simulink model "RM3_Hydraulic_PTO_NEW"  (R2019b)
settings: Solver=ode14x  StartTime=0  StopTime=200  FixedStep=0.0025  MaxStep=0.0025  RelTol=1e-3  EnableMultiTasking=on
undefined symbols (not defined in the file or in its folder): body, DiscIntNeverNeededParam, pto
libraries: fl_lib x1519, nesl_utility x807, sh_lib x675, WECSim_Lib x5
(part 2 of 56)

== system RM3_Hydraulic_PTO_NEW/PTO-Sim - Crankshaft DA 4 Cylinders Case 2 extra ==
  response : Inport
  " Flow Rate Accum Sensor" : fl_lib/Hydraulic/Hydraulic Sensors/Hydraulic Flow Rate Sensor  Commented=on
      settings: SourceProductName=Simscape
  1000 psi Pressure Relief Valve : sh_lib/Valves/Pressure Control Valves/Pressure Relief Valve  valve_area_spec=1  p_diff_TLU=[30.15e5 : 15e3 : 31.35e5] Pa  area_TLU=[1 : 1 : 9] .* 1e-5 m^2  area_max=pi*(0.75/2)^2 in^2  pres_set=1000 psi  reg_range=50 psi  C_d=0.7  A_leak=1e-12 m^2  lam_spec=1  B_lam=0.999  Re_cr=12  dynamic=0  tau=0.1 s  area_init=1e-12 m^2
      settings: SourceProductName=Simscape Fluids  SourceProductBaseCode=SH  InternalSimscapePortConfiguration="{\"Bottom\":[],\"Left\":[{\"id\":\"A\",\"label\":\"A\",\"type\":\"foundation.hydraulic.hydraulic\"}],\"Right\":[{\"id\":\"B\",\"label\":\"B\",\"type\":\"foundation.hydraulic.hydraulic\"}],\"Top\":[]}"
  Accumulator Volume Scope : Scope  Commented=on
  Ang Velocity signal : Product  Inputs=*/
  Bus Selector : BusSelector  OutputSignals=position,velocity
  Constant1 : Constant  Value=0
  Crank Initial Angle (rad) 1 : Constant  Value=pi/2
  Crank Initial Angle (rad) 2 : Constant  Value=0
  Crank Initial Angle (rad) 3 : Constant  Value=3*pi/2
  Crank Initial Angle (rad) 4 : Constant  Value=pi
  Crank Radius (m) : Constant  Value=0.1397
  Cylinder 1 : Subsystem
  Cylinder 2 : Subsystem
  Cylinder 3 : Subsystem
  Cylinder 4 : Subsystem
  Delay1 : Delay  Commented=on  DelayLength=1
  Delay2 : Delay  DelayLength=1
  Discrete-Time Integrator : DiscreteIntegrator  Commented=on  SampleTime=-1  ICPrevOutput=DiscIntNeverNeededParam  ICPrevScaledInput=DiscIntNeverNeededParam
  Discrete-Time Integrator - Angle Disp : DiscreteIntegrator  SampleTime=-1  ICPrevOutput=DiscIntNeverNeededParam  ICPrevScaledInput=DiscIntNeverNeededParam
  Gain : Gain  Commented=on
  Gain1 : Gain  Commented=on  Gain=-11000
  Gas-Charged Accumulator : sh_lib/Accumulators/Gas-Charged Accumulator  Commented=on  capacity=2.5 gal  dead_volume=4e-5 m^3  pr_preload=800 psi  k_sh=1.4  stiff_coeff=1e10 Pa/m^3  penetr_coeff=1e10 s*Pa/m^6  flow_rate_specify=off  flow_rate_priority=None  flow_rate=0.005 m^3/s  flow_rate_nominal_specify=off  flow_rate_nominal_unit=m^3/s  flow_rate_nominal_value=1  liquid_volume_specify=on  liquid_volume_priority=High  liquid_volume=0.005 m^3  liquid_volume_nominal_specify=off  liquid_volume_nominal_unit=m^3  liquid_volume_nominal_value=1  liquid_pressure_specify=off  liquid_pressure_priority=None  liquid_pressure=1.01325e+5 Pa  liquid_pressure_nominal_specify=off  liquid_pressure_nominal_unit=Pa  liquid_pressure_nominal_value=1
      settings: SourceProductName=Simscape Fluids  SourceProductBaseCode=SH  InternalSimscapePortConfiguration="{\"Bottom\":[],\"Left\":[],\"Right\":[{\"id\":\"A\",\"label\":\"A\",\"type\":\"foundation.hydraulic.hydraulic\"}],\"Top\":[]}"
  Hydraulic Reference : fl_lib/Hydraulic/Hydraulic Elements/Hydraulic Reference
      settings: SourceProductName=Simscape
  Ideal Angular Velocity Source : fl_lib/Mechanical/Mechanical Sources/Ideal Angular Velocity Source
  Linear Position Scope : Scope
  Linear Velocity Scope : Scope
  Mechanical Rotational Reference : fl_lib/Mechanical/Rotational Elements/Mechanical Rotational Reference
  Mux : Mux  Inputs=10
  Mux1 : Mux  Inputs=3
  Ocean Intake (5m depth) : fl_lib/Hydraulic/Hydraulic Elements/Hydraulic Reference
      settings: SourceProductName=Simscape
  PS-Simulink Converter : nesl_utility/PS-Simulink Converter  Commented=on  PhysicalDomain=network_engine_domain  SubClassName=ps_output  LeftPortType=input  RightPortType=output  PseudoPeriodic=off  Frequencies=[]  Unit=inherit  AffineConversion=off
  PS-Simulink Converter{1..10} (10 alike) : nesl_utility/PS-Simulink Converter  PhysicalDomain=network_engine_domain  SubClassName=ps_output  LeftPortType=input  RightPortType=output  PseudoPeriodic=off  Frequencies=[]  Unit=inherit  AffineConversion=off
  Plus : Sum  Commented=on
  "Point of zero spring force (submerged distance) " : Constant  Value=4
  Pressure Sensor RV : fl_lib/Hydraulic/Hydraulic Sensors/Hydraulic Pressure Sensor
      settings: SourceProductName=Simscape
  Product : Product
  RO Membrane : Subsystem
  Sea Water : sh_lib/Hydraulic Utilities/Hydraulic Fluid  DataSource=1  SelFluid=24  SysTemp=30  TrapAir=0.005  ViscDerFactor=1  range_error=2
      settings: SourceProductName=Simscape Fluids
  Selector : Selector  InputPortWidth=6  IndexOptions=Index vector (dialog)  Indices=3  OutputSizes=1
  Selector1 : Selector  InputPortWidth=6  IndexOptions=Index vector (dialog)  Indices=3  OutputSizes=1
  Simulink-PS Converter : nesl_utility/Simulink-PS Converter  PhysicalDomain=network_engine_domain  SubClassName=ps_input  LeftPortType=input  RightPortType=output  PseudoPeriodic=off  Frequencies=[]  NoiseDistribution=none  NoiseParameters=[]  Unit=rad/s  AffineConversion=off  FilteringAndDerivatives=filter  SimscapeFilterOrder=2  InputFilterTimeConstant=0.001  UdotUserProvided=0
  Sine Wave2 : Sin  Commented=on  Amplitude=0.45  Frequency=0.9  SampleTime=0.01
  Solver Configuration : nesl_utility/Solver Configuration  PhysicalDomain=network_engine_domain  SubClassName=solver  LeftPortType=input  RightPortType=generic  Tones=[]  Harmonics=[]  SimulateNoise=off  Profile=off  UseLocalSampling=off  EnableSwitchedLinearOptims=on  FrequencyDomain=off  UseCCode=off  RelTol=0.001  AbsTol=1e-06  MinStep=1e-09  ToWorkspace=off  RevertToSquareIcSolve=off  NumHomotopyIterations=100  PhasorMode=off  PhasorModeNumHarmonics=1  DoDC=off  ResidualTolerance=1e-09  UseLocalSolver=off  LocalSolverChoice=NE_BACKWARD_EULER_ADVANCER  LocalSolverSampleTime=0.001  DoFixedCost=off  MaxNonlinIter=3  MaxModeIter=2  LinearAlgebra=auto  EquationFormulation=NE_TIME_EF  DelaysMemoryBudget=1024  AutomaticFiltering=on  FilteringTimeConstant=0.01  PartitionStorageMethod=AS_NEEDED  PartitionMemoryBudget=1024  PartitionMethod=ROBUST
  Spool Radius (m) : Constant  Value=0.1397
  Spring Constant : Gain  Gain=-200
  Spring Constant1 : Gain  Commented=on  Gain=840
  Spring Constant2 : Gain  Commented=on  Gain=-400
  Sum : Sum  Inputs=|++
  Sum1 : Sum  Inputs=|++
  Sum2 : Sum  Inputs=4
  Switch : Switch  Criteria=u2 > Threshold
  Terminator : Terminator
  To Workspace : ToWorkspace  VariableName=output_RO  SaveFormat=Structure With Time  SampleTime=-1
  To Workspace1 : ToWorkspace  VariableName=output_Power  SaveFormat=Structure With Time  SampleTime=-1
  Water Quality Block : Subsystem
  Forces : Outport  VectorParamsAs1DForOutWhenUnconnected=off
  wires:
  Bus Selector/1 -> Selector/1  "<position>"
  Bus Selector/2 -> Selector1/1  "<velocity>"
  response/1 -> Bus Selector/1
  Selector/1 -> Linear Position Scope/1, Sum1/1, Terminator/1
  Spring Constant/1 -> Sum/2
  Gain1/1 -> Plus/2
  Sum/1 -> Delay2/1
  Constant1/1 -> Switch/3
  Switch/1 -> Ang Velocity signal/1
  Selector1/1 -> Linear Velocity Scope/1, Mux1/3, Product/1, Switch/2, Switch/1  "V_linear"
  Ang Velocity signal/1 -> Discrete-Time Integrator - Angle Disp/1, Simulink-PS Converter/1
  "Point of zero spring force (submerged distance) "/1 -> Sum1/2
  Sum1/1 -> Spring Constant/1
  Delay2/1 -> Product/2, Mux1/1, Forces/1  "Force"
  PS-Simulink Converter/1 -> Discrete-Time Integrator/1
  Discrete-Time Integrator/1 -> Accumulator Volume Scope/1
  Crank Radius (m)/1 -> Cylinder 4/1(Crank Radius), Cylinder 3/1(Crank Radius), Cylinder 2/1(Crank Radius), Cylinder 1/1(Crank Radius)
  Discrete-Time Integrator - Angle Disp/1 -> Cylinder 4/3(Angle Displacement), Cylinder 3/3(Angle Displacement), Cylinder 2/3(Angle Displacement), Cylinder 1/3(Angle Displacement)
  Crank Initial Angle (rad) 1/1 -> Cylinder 1/4(Crank Init Angle)
  Sum2/1 -> Sum/1
  Cylinder 1/1(PTO Force) -> Sum2/4
  Cylinder 2/1(PTO Force) -> Sum2/3
  Cylinder 3/1(PTO Force) -> Sum2/2
  Cylinder 4/1(PTO Force) -> Sum2/1
  Spool Radius (m)/1 -> Cylinder 1/2(Spool Radius), Cylinder 4/2(Spool Radius), Cylinder 3/2(Spool Radius), Cylinder 2/2(Spool Radius), Ang Velocity signal/2
  Crank Initial Angle (rad) 4/1 -> Cylinder 4/4(Crank Init Angle)
  Crank Initial Angle (rad) 3/1 -> Cylinder 3/4(Crank Init Angle)
  Crank Initial Angle (rad) 2/1 -> Cylinder 2/4(Crank Init Angle)
  PS-Simulink Converter6/1 -> Mux/7  "Feed Mass Flow Rate"
  PS-Simulink Converter10/1 -> Mux/6  "Brine Mass Flow Rate"
  PS-Simulink Converter9/1 -> Mux/9  "Brine Flow Rate"
  PS-Simulink Converter8/1 -> Mux/8  "Permeate Mass Flow Rate"
  Mux/1 -> To Workspace/1
  PS-Simulink Converter4/1 -> Mux/4  "Permeate Flow Rate"
  PS-Simulink Converter1/1 -> Mux/1  "P before RO after OSM"
  PS-Simulink Converter2/1 -> Mux/2  "P drop RO"
  PS-Simulink Converter3/1 -> Mux/3  "Feed Flow Rate"
  PS-Simulink Converter5/1 -> Mux/5  "Feed Pressure"
  PS-Simulink Converter7/1 -> Mux/10  "Pressure Brine Exit"
  Mux1/1 -> To Workspace1/1
  Product/1 -> Mux1/2  "Power"
  connections:
  Solver Configuration/RConn1 -- Ocean Intake (5m depth)/LConn1 -- Sea Water/RConn1 -- Cylinder 4/LConn3 -- Cylinder 3/LConn3 -- Cylinder 2/LConn3 -- Cylinder 1/LConn3
  Ideal Angular Velocity Source/RConn2 -- Mechanical Rotational Reference/LConn1
  Ideal Angular Velocity Source/RConn1 -- Simulink-PS Converter/RConn1
  1000 psi Pressure Relief Valve/RConn1 -- Pressure Sensor RV/RConn1 -- Hydraulic Reference/LConn1
  Gas-Charged Accumulator/RConn1 -- Cylinder 1/LConn2 -- Cylinder 3/LConn2 -- Cylinder 4/LConn2 -- Cylinder 2/LConn2 -- RO Membrane/LConn1 -- 1000 psi Pressure Relief Valve/LConn1 -- Pressure Sensor RV/LConn1
  " Flow Rate Accum Sensor"/RConn1 -- PS-Simulink Converter/LConn1
  Cylinder 1/LConn1 -- Cylinder 2/LConn1 -- Cylinder 3/LConn1 -- Cylinder 4/LConn1 -- Ideal Angular Velocity Source/LConn1
  PS-Simulink Converter10/LConn1 -- RO Membrane/RConn9
  PS-Simulink Converter3/LConn1 -- RO Membrane/RConn3 -- Water Quality Block/LConn3
  PS-Simulink Converter9/LConn1 -- RO Membrane/RConn8
  PS-Simulink Converter1/LConn1 -- RO Membrane/RConn1 -- Water Quality Block/LConn1
  PS-Simulink Converter8/LConn1 -- RO Membrane/RConn7
  PS-Simulink Converter6/LConn1 -- RO Membrane/RConn6
  RO Membrane/RConn4 -- PS-Simulink Converter4/LConn1 -- Water Quality Block/LConn4
  PS-Simulink Converter2/LConn1 -- RO Membrane/RConn2 -- Water Quality Block/LConn2
  RO Membrane/RConn5 -- PS-Simulink Converter5/LConn1
  PS-Simulink Converter7/LConn1 -- RO Membrane/RConn10

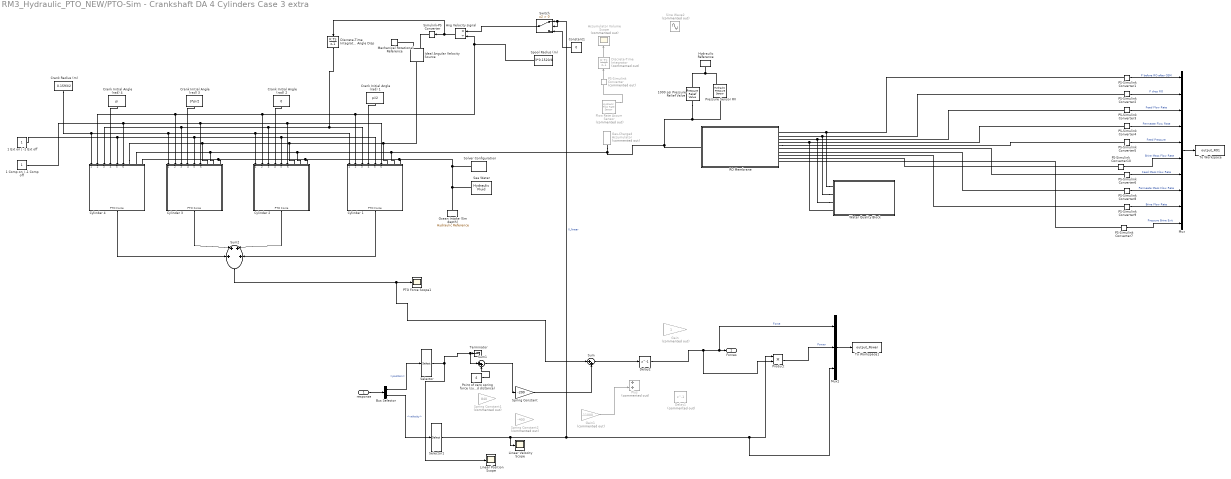
== system RM3_Hydraulic_PTO_NEW/PTO-Sim - Crankshaft DA 4 Cylinders Case 3 extra ==
  response : Inport
  " Flow Rate Accum Sensor" : fl_lib/Hydraulic/Hydraulic Sensors/Hydraulic Flow Rate Sensor  Commented=on
      settings: SourceProductName=Simscape
  1 Comp on | -1 Comp off : Constant
  1 Ext on | -1 Ext off : Constant
  1000 psi Pressure Relief Valve : sh_lib/Valves/Pressure Control Valves/Pressure Relief Valve  valve_area_spec=1  p_diff_TLU=[30.15e5 : 15e3 : 31.35e5] Pa  area_TLU=[1 : 1 : 9] .* 1e-5 m^2  area_max=pi*(0.75/2)^2 in^2  pres_set=1000 psi  reg_range=50 psi  C_d=0.7  A_leak=1e-12 m^2  lam_spec=1  B_lam=0.999  Re_cr=12  dynamic=0  tau=0.1 s  area_init=1e-12 m^2
      settings: SourceProductName=Simscape Fluids  SourceProductBaseCode=SH  InternalSimscapePortConfiguration="{\"Bottom\":[],\"Left\":[{\"id\":\"A\",\"label\":\"A\",\"type\":\"foundation.hydraulic.hydraulic\"}],\"Right\":[{\"id\":\"B\",\"label\":\"B\",\"type\":\"foundation.hydraulic.hydraulic\"}],\"Top\":[]}"
  Accumulator Volume Scope : Scope  Commented=on
  Ang Velocity signal : Product  Inputs=*/
  Bus Selector : BusSelector  OutputSignals=position,velocity
  Constant1 : Constant  Value=0
  Crank Initial Angle (rad) 1 : Constant  Value=pi/2
  Crank Initial Angle (rad) 2 : Constant  Value=0
  Crank Initial Angle (rad) 3 : Constant  Value=3*pi/2
  Crank Initial Angle (rad) 4 : Constant  Value=pi
  Crank Radius (m) : Constant  Value=0.1593/2
  Cylinder 1 : Subsystem
  Cylinder 2 : Subsystem
  Cylinder 3 : Subsystem
  Cylinder 4 : Subsystem
  Delay1 : Delay  Commented=on  DelayLength=1
  Delay2 : Delay  DelayLength=1
  Discrete-Time Integrator : DiscreteIntegrator  Commented=on  SampleTime=-1  ICPrevOutput=DiscIntNeverNeededParam  ICPrevScaledInput=DiscIntNeverNeededParam
  Discrete-Time Integrator - Angle Disp : DiscreteIntegrator  SampleTime=-1  ICPrevOutput=DiscIntNeverNeededParam  ICPrevScaledInput=DiscIntNeverNeededParam
  Gain : Gain  Commented=on
  Gain1 : Gain  Commented=on  Gain=-11000
  Gas-Charged Accumulator : sh_lib/Accumulators/Gas-Charged Accumulator  Commented=on  capacity=2.5 gal  dead_volume=4e-5 m^3  pr_preload=800 psi  k_sh=1.4  stiff_coeff=1e10 Pa/m^3  penetr_coeff=1e10 s*Pa/m^6  flow_rate_specify=off  flow_rate_priority=None  flow_rate=0.005 m^3/s  flow_rate_nominal_specify=off  flow_rate_nominal_unit=m^3/s  flow_rate_nominal_value=1  liquid_volume_specify=on  liquid_volume_priority=High  liquid_volume=0.005 m^3  liquid_volume_nominal_specify=off  liquid_volume_nominal_unit=m^3  liquid_volume_nominal_value=1  liquid_pressure_specify=off  liquid_pressure_priority=None  liquid_pressure=1.01325e+5 Pa  liquid_pressure_nominal_specify=off  liquid_pressure_nominal_unit=Pa  liquid_pressure_nominal_value=1
      settings: SourceProductName=Simscape Fluids  SourceProductBaseCode=SH  InternalSimscapePortConfiguration="{\"Bottom\":[],\"Left\":[],\"Right\":[{\"id\":\"A\",\"label\":\"A\",\"type\":\"foundation.hydraulic.hydraulic\"}],\"Top\":[]}"
  Hydraulic Reference : fl_lib/Hydraulic/Hydraulic Elements/Hydraulic Reference
      settings: SourceProductName=Simscape
  Ideal Angular Velocity Source : fl_lib/Mechanical/Mechanical Sources/Ideal Angular Velocity Source
  Linear Position Scope : Scope
  Linear Velocity Scope : Scope
  Mechanical Rotational Reference : fl_lib/Mechanical/Rotational Elements/Mechanical Rotational Reference
  Mux : Mux  Inputs=10
  Mux1 : Mux  Inputs=3
  Ocean Intake (5m depth) : fl_lib/Hydraulic/Hydraulic Elements/Hydraulic Reference
      settings: SourceProductName=Simscape
  PS-Simulink Converter : nesl_utility/PS-Simulink Converter  Commented=on  PhysicalDomain=network_engine_domain  SubClassName=ps_output  LeftPortType=input  RightPortType=output  PseudoPeriodic=off  Frequencies=[]  Unit=inherit  AffineConversion=off
  PS-Simulink Converter{1..10} (10 alike) : nesl_utility/PS-Simulink Converter  PhysicalDomain=network_engine_domain  SubClassName=ps_output  LeftPortType=input  RightPortType=output  PseudoPeriodic=off  Frequencies=[]  Unit=inherit  AffineConversion=off
  PTO Force Scope1 : Scope
  Plus : Sum  Commented=on
  "Point of zero spring force (submerged distance) " : Constant  Value=4
  Pressure Sensor RV : fl_lib/Hydraulic/Hydraulic Sensors/Hydraulic Pressure Sensor
      settings: SourceProductName=Simscape
  Product : Product
  RO Membrane : Subsystem
  Sea Water : sh_lib/Hydraulic Utilities/Hydraulic Fluid  DataSource=1  SelFluid=24  SysTemp=30  TrapAir=0.005  ViscDerFactor=1  range_error=2
      settings: SourceProductName=Simscape Fluids
  Selector : Selector  InputPortWidth=6  IndexOptions=Index vector (dialog)  Indices=3  OutputSizes=1
  Selector1 : Selector  InputPortWidth=6  IndexOptions=Index vector (dialog)  Indices=3  OutputSizes=1
  Simulink-PS Converter : nesl_utility/Simulink-PS Converter  PhysicalDomain=network_engine_domain  SubClassName=ps_input  LeftPortType=input  RightPortType=output  PseudoPeriodic=off  Frequencies=[]  NoiseDistribution=none  NoiseParameters=[]  Unit=rad/s  AffineConversion=off  FilteringAndDerivatives=filter  SimscapeFilterOrder=2  InputFilterTimeConstant=0.001  UdotUserProvided=0
  Sine Wave2 : Sin  Commented=on  Amplitude=0.45/4  Frequency=0.9  SampleTime=0.01
  Solver Configuration : nesl_utility/Solver Configuration  PhysicalDomain=network_engine_domain  SubClassName=solver  LeftPortType=input  RightPortType=generic  Tones=[]  Harmonics=[]  SimulateNoise=off  Profile=off  UseLocalSampling=off  EnableSwitchedLinearOptims=on  FrequencyDomain=off  UseCCode=off  RelTol=0.001  AbsTol=1e-06  MinStep=1e-09  ToWorkspace=off  RevertToSquareIcSolve=off  NumHomotopyIterations=100  PhasorMode=off  PhasorModeNumHarmonics=1  DoDC=off  ResidualTolerance=1e-09  UseLocalSolver=off  LocalSolverChoice=NE_BACKWARD_EULER_ADVANCER  LocalSolverSampleTime=0.001  DoFixedCost=off  MaxNonlinIter=3  MaxModeIter=2  LinearAlgebra=auto  EquationFormulation=NE_TIME_EF  DelaysMemoryBudget=1024  AutomaticFiltering=on  FilteringTimeConstant=0.01  PartitionStorageMethod=AS_NEEDED  PartitionMemoryBudget=1024  PartitionMethod=ROBUST
  Spool Radius (m) : Constant  Value=3*0.1520/4
  Spring Constant : Gain  Gain=-200
  Spring Constant1 : Gain  Commented=on  Gain=840
  Spring Constant2 : Gain  Commented=on  Gain=-400
  Sum : Sum  Inputs=|++
  Sum1 : Sum  Inputs=|++
  Sum2 : Sum  Inputs=4
  Switch : Switch  Criteria=u2 > Threshold
  Terminator : Terminator
  To Workspace : ToWorkspace  VariableName=output_RO1  SaveFormat=Structure With Time  SampleTime=-1
  To Workspace1 : ToWorkspace  VariableName=output_Power  SaveFormat=Structure With Time  SampleTime=-1
  Water Quality Block : Subsystem
  Forces : Outport  VectorParamsAs1DForOutWhenUnconnected=off
  wires:
  Bus Selector/1 -> Selector/1  "<position>"
  Bus Selector/2 -> Selector1/1  "<velocity>"
  response/1 -> Bus Selector/1
  Selector/1 -> Linear Position Scope/1, Sum1/1, Terminator/1
  Spring Constant/1 -> Sum/2
  Gain1/1 -> Plus/2
  Sum/1 -> Delay2/1
  Selector1/1 -> Linear Velocity Scope/1, Mux1/3, Product/1, Switch/2, Switch/1  "V_linear"
  "Point of zero spring force (submerged distance) "/1 -> Sum1/2
  Sum1/1 -> Spring Constant/1
  Delay2/1 -> Product/2, Mux1/1, Forces/1  "Force"
  Mux1/1 -> To Workspace1/1
  Product/1 -> Mux1/2  "Power"
  1 Ext on | -1 Ext off/1 -> Cylinder 1/5(Ext Control Input), Cylinder 2/5(Ext Control Input), Cylinder 3/5(Ext Control Input), Cylinder 4/5(Ext Control Input)
  1 Comp on | -1 Comp off/1 -> Cylinder 1/6(Comp Control Input), Cylinder 2/6(Comp Control Input), Cylinder 3/6(Comp Control Input), Cylinder 4/6(Comp Control Input)
  Sum2/1 -> PTO Force Scope1/1, Sum/1
  PS-Simulink Converter7/1 -> Mux/10  "Pressure Brine Exit"
  Discrete-Time Integrator/1 -> Accumulator Volume Scope/1
  PS-Simulink Converter/1 -> Discrete-Time Integrator/1
  PS-Simulink Converter9/1 -> Mux/9  "Brine Flow Rate"
  PS-Simulink Converter5/1 -> Mux/5  "Feed Pressure"
  Cylinder 1/1(PTO Force) -> Sum2/4
  PS-Simulink Converter8/1 -> Mux/8  "Permeate Mass Flow Rate"
  PS-Simulink Converter10/1 -> Mux/6  "Brine Mass Flow Rate"
  PS-Simulink Converter6/1 -> Mux/7  "Feed Mass Flow Rate"
  PS-Simulink Converter4/1 -> Mux/4  "Permeate Flow Rate"
  PS-Simulink Converter1/1 -> Mux/1  "P before RO after OSM"
  Constant1/1 -> Switch/3
  Mux/1 -> To Workspace/1
  Cylinder 2/1(PTO Force) -> Sum2/3
  Crank Radius (m)/1 -> Cylinder 1/1(Crank Radius), Cylinder 2/1(Crank Radius), Cylinder 3/1(Crank Radius), Cylinder 4/1(Crank Radius)
  PS-Simulink Converter2/1 -> Mux/2  "P drop RO"
  Ang Velocity signal/1 -> Discrete-Time Integrator - Angle Disp/1, Simulink-PS Converter/1
  Spool Radius (m)/1 -> Cylinder 1/2(Spool Radius), Cylinder 4/2(Spool Radius), Cylinder 3/2(Spool Radius), Cylinder 2/2(Spool Radius), Ang Velocity signal/2
  Discrete-Time Integrator - Angle Disp/1 -> Cylinder 4/3(Angle Displacement), Cylinder 3/3(Angle Displacement), Cylinder 2/3(Angle Displacement), Cylinder 1/3(Angle Displacement)
  Cylinder 4/1(PTO Force) -> Sum2/1
  Crank Initial Angle (rad) 3/1 -> Cylinder 3/4(Crank Init Angle)
  Crank Initial Angle (rad) 2/1 -> Cylinder 2/4(Crank Init Angle)
  Crank Initial Angle (rad) 1/1 -> Cylinder 1/4(Crank Init Angle)
  Cylinder 3/1(PTO Force) -> Sum2/2
  Switch/1 -> Ang Velocity signal/1
  Crank Initial Angle (rad) 4/1 -> Cylinder 4/4(Crank Init Angle)
  PS-Simulink Converter3/1 -> Mux/3  "Feed Flow Rate"
  connections:
  Hydraulic Reference/LConn1 -- 1000 psi Pressure Relief Valve/RConn1 -- Pressure Sensor RV/RConn1
  Water Quality Block/LConn4 -- RO Membrane/RConn4 -- PS-Simulink Converter4/LConn1
  Water Quality Block/LConn1 -- PS-Simulink Converter1/LConn1 -- RO Membrane/RConn1
  Cylinder 4/LConn1 -- Cylinder 3/LConn1 -- Cylinder 1/LConn1 -- Ideal Angular Velocity Source/LConn1 -- Cylinder 2/LConn1
  Water Quality Block/LConn3 -- PS-Simulink Converter3/LConn1 -- RO Membrane/RConn3
  Cylinder 1/LConn3 -- Cylinder 4/LConn3 -- Cylinder 3/LConn3 -- Cylinder 2/LConn3 -- Solver Configuration/RConn1 -- Ocean Intake (5m depth)/LConn1 -- Sea Water/RConn1
  Pressure Sensor RV/LConn1 -- 1000 psi Pressure Relief Valve/LConn1 -- RO Membrane/LConn1 -- Gas-Charged Accumulator/RConn1 -- Cylinder 1/LConn2 -- Cylinder 3/LConn2 -- Cylinder 4/LConn2 -- Cylinder 2/LConn2
  Water Quality Block/LConn2 -- PS-Simulink Converter2/LConn1 -- RO Membrane/RConn2
  PS-Simulink Converter10/LConn1 -- RO Membrane/RConn9
  PS-Simulink Converter8/LConn1 -- RO Membrane/RConn7
  PS-Simulink Converter7/LConn1 -- RO Membrane/RConn10
  RO Membrane/RConn5 -- PS-Simulink Converter5/LConn1
  Ideal Angular Velocity Source/RConn1 -- Simulink-PS Converter/RConn1
  PS-Simulink Converter9/LConn1 -- RO Membrane/RConn8
  PS-Simulink Converter6/LConn1 -- RO Membrane/RConn6
  Ideal Angular Velocity Source/RConn2 -- Mechanical Rotational Reference/LConn1
  " Flow Rate Accum Sensor"/RConn1 -- PS-Simulink Converter/LConn1

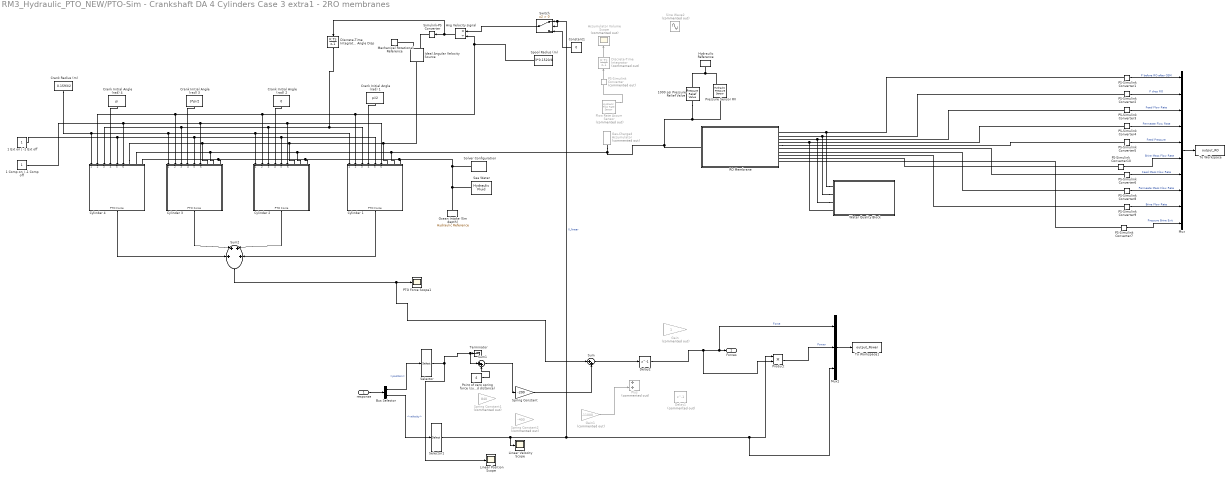
== system RM3_Hydraulic_PTO_NEW/PTO-Sim - Crankshaft DA 4 Cylinders Case 3 extra1 - 2RO membranes ==
  response : Inport
  " Flow Rate Accum Sensor" : fl_lib/Hydraulic/Hydraulic Sensors/Hydraulic Flow Rate Sensor  Commented=on
      settings: SourceProductName=Simscape
  1 Comp on | -1 Comp off : Constant
  1 Ext on | -1 Ext off : Constant
  1000 psi Pressure Relief Valve : sh_lib/Valves/Pressure Control Valves/Pressure Relief Valve  valve_area_spec=1  p_diff_TLU=[30.15e5 : 15e3 : 31.35e5] Pa  area_TLU=[1 : 1 : 9] .* 1e-5 m^2  area_max=pi*(0.75/2)^2 in^2  pres_set=1000 psi  reg_range=50 psi  C_d=0.7  A_leak=1e-12 m^2  lam_spec=1  B_lam=0.999  Re_cr=12  dynamic=0  tau=0.1 s  area_init=1e-12 m^2
      settings: SourceProductName=Simscape Fluids  SourceProductBaseCode=SH  InternalSimscapePortConfiguration="{\"Bottom\":[],\"Left\":[{\"id\":\"A\",\"label\":\"A\",\"type\":\"foundation.hydraulic.hydraulic\"}],\"Right\":[{\"id\":\"B\",\"label\":\"B\",\"type\":\"foundation.hydraulic.hydraulic\"}],\"Top\":[]}"
  Accumulator Volume Scope : Scope  Commented=on
  Ang Velocity signal : Product  Inputs=*/
  Bus Selector : BusSelector  OutputSignals=position,velocity
  Constant1 : Constant  Value=0
  Crank Initial Angle (rad) 1 : Constant  Value=pi/2
  Crank Initial Angle (rad) 2 : Constant  Value=0
  Crank Initial Angle (rad) 3 : Constant  Value=3*pi/2
  Crank Initial Angle (rad) 4 : Constant  Value=pi
  Crank Radius (m) : Constant  Value=0.1593/2
  Cylinder 1 : Subsystem
  Cylinder 2 : Subsystem
  Cylinder 3 : Subsystem
  Cylinder 4 : Subsystem
  Delay1 : Delay  Commented=on  DelayLength=1
  Delay2 : Delay  DelayLength=1
  Discrete-Time Integrator : DiscreteIntegrator  Commented=on  SampleTime=-1  ICPrevOutput=DiscIntNeverNeededParam  ICPrevScaledInput=DiscIntNeverNeededParam
  Discrete-Time Integrator - Angle Disp : DiscreteIntegrator  SampleTime=-1  ICPrevOutput=DiscIntNeverNeededParam  ICPrevScaledInput=DiscIntNeverNeededParam
  Gain : Gain  Commented=on
  Gain1 : Gain  Commented=on  Gain=-11000
  Gas-Charged Accumulator : sh_lib/Accumulators/Gas-Charged Accumulator  Commented=on  capacity=2.5 gal  dead_volume=4e-5 m^3  pr_preload=800 psi  k_sh=1.4  stiff_coeff=1e10 Pa/m^3  penetr_coeff=1e10 s*Pa/m^6  flow_rate_specify=off  flow_rate_priority=None  flow_rate=0.005 m^3/s  flow_rate_nominal_specify=off  flow_rate_nominal_unit=m^3/s  flow_rate_nominal_value=1  liquid_volume_specify=on  liquid_volume_priority=High  liquid_volume=0.005 m^3  liquid_volume_nominal_specify=off  liquid_volume_nominal_unit=m^3  liquid_volume_nominal_value=1  liquid_pressure_specify=off  liquid_pressure_priority=None  liquid_pressure=1.01325e+5 Pa  liquid_pressure_nominal_specify=off  liquid_pressure_nominal_unit=Pa  liquid_pressure_nominal_value=1
      settings: SourceProductName=Simscape Fluids  SourceProductBaseCode=SH  InternalSimscapePortConfiguration="{\"Bottom\":[],\"Left\":[],\"Right\":[{\"id\":\"A\",\"label\":\"A\",\"type\":\"foundation.hydraulic.hydraulic\"}],\"Top\":[]}"
  Hydraulic Reference : fl_lib/Hydraulic/Hydraulic Elements/Hydraulic Reference
      settings: SourceProductName=Simscape
  Ideal Angular Velocity Source : fl_lib/Mechanical/Mechanical Sources/Ideal Angular Velocity Source
  Linear Position Scope : Scope
  Linear Velocity Scope : Scope
  Mechanical Rotational Reference : fl_lib/Mechanical/Rotational Elements/Mechanical Rotational Reference
  Mux : Mux  Inputs=10
  Mux1 : Mux  Inputs=3
  Ocean Intake (5m depth) : fl_lib/Hydraulic/Hydraulic Elements/Hydraulic Reference
      settings: SourceProductName=Simscape
  PS-Simulink Converter : nesl_utility/PS-Simulink Converter  Commented=on  PhysicalDomain=network_engine_domain  SubClassName=ps_output  LeftPortType=input  RightPortType=output  PseudoPeriodic=off  Frequencies=[]  Unit=inherit  AffineConversion=off
  PS-Simulink Converter{1..10} (10 alike) : nesl_utility/PS-Simulink Converter  PhysicalDomain=network_engine_domain  SubClassName=ps_output  LeftPortType=input  RightPortType=output  PseudoPeriodic=off  Frequencies=[]  Unit=inherit  AffineConversion=off
  PTO Force Scope1 : Scope
  Plus : Sum  Commented=on
  "Point of zero spring force (submerged distance) " : Constant  Value=4
  Pressure Sensor RV : fl_lib/Hydraulic/Hydraulic Sensors/Hydraulic Pressure Sensor
      settings: SourceProductName=Simscape
  Product : Product
  RO Membrane : Subsystem
  Sea Water : sh_lib/Hydraulic Utilities/Hydraulic Fluid  DataSource=1  SelFluid=24  SysTemp=30  TrapAir=0.005  ViscDerFactor=1  range_error=2
      settings: SourceProductName=Simscape Fluids
  Selector : Selector  InputPortWidth=6  IndexOptions=Index vector (dialog)  Indices=3  OutputSizes=1
  Selector1 : Selector  InputPortWidth=6  IndexOptions=Index vector (dialog)  Indices=3  OutputSizes=1
  Simulink-PS Converter : nesl_utility/Simulink-PS Converter  PhysicalDomain=network_engine_domain  SubClassName=ps_input  LeftPortType=input  RightPortType=output  PseudoPeriodic=off  Frequencies=[]  NoiseDistribution=none  NoiseParameters=[]  Unit=rad/s  AffineConversion=off  FilteringAndDerivatives=filter  SimscapeFilterOrder=2  InputFilterTimeConstant=0.001  UdotUserProvided=0
  Sine Wave2 : Sin  Commented=on  Amplitude=0.45/4  Frequency=0.9  SampleTime=0.01
  Solver Configuration : nesl_utility/Solver Configuration  PhysicalDomain=network_engine_domain  SubClassName=solver  LeftPortType=input  RightPortType=generic  Tones=[]  Harmonics=[]  SimulateNoise=off  Profile=off  UseLocalSampling=off  EnableSwitchedLinearOptims=on  FrequencyDomain=off  UseCCode=off  RelTol=0.001  AbsTol=1e-06  MinStep=1e-09  ToWorkspace=off  RevertToSquareIcSolve=off  NumHomotopyIterations=100  PhasorMode=off  PhasorModeNumHarmonics=1  DoDC=off  ResidualTolerance=1e-09  UseLocalSolver=off  LocalSolverChoice=NE_BACKWARD_EULER_ADVANCER  LocalSolverSampleTime=0.001  DoFixedCost=off  MaxNonlinIter=3  MaxModeIter=2  LinearAlgebra=auto  EquationFormulation=NE_TIME_EF  DelaysMemoryBudget=1024  AutomaticFiltering=on  FilteringTimeConstant=0.01  PartitionStorageMethod=AS_NEEDED  PartitionMemoryBudget=1024  PartitionMethod=ROBUST
  Spool Radius (m) : Constant  Value=3*0.1520/4
  Spring Constant : Gain  Gain=-200
  Spring Constant1 : Gain  Commented=on  Gain=840
  Spring Constant2 : Gain  Commented=on  Gain=-400
  Sum : Sum  Inputs=|++
  Sum1 : Sum  Inputs=|++
  Sum2 : Sum  Inputs=4
  Switch : Switch  Criteria=u2 > Threshold
  Terminator : Terminator
  To Workspace : ToWorkspace  VariableName=output_RO  SaveFormat=Structure With Time  SampleTime=-1
  To Workspace1 : ToWorkspace  VariableName=output_Power  SaveFormat=Structure With Time  SampleTime=-1
  Water Quality Block : Subsystem
  Forces : Outport  VectorParamsAs1DForOutWhenUnconnected=off
  wires:
  Bus Selector/1 -> Selector/1  "<position>"
  Bus Selector/2 -> Selector1/1  "<velocity>"
  response/1 -> Bus Selector/1
  Selector/1 -> Linear Position Scope/1, Sum1/1, Terminator/1
  Spring Constant/1 -> Sum/2
  Gain1/1 -> Plus/2
  Sum/1 -> Delay2/1
  Selector1/1 -> Linear Velocity Scope/1, Mux1/3, Product/1, Switch/2, Switch/1  "V_linear"
  "Point of zero spring force (submerged distance) "/1 -> Sum1/2
  Sum1/1 -> Spring Constant/1
  Delay2/1 -> Product/2, Mux1/1, Forces/1  "Force"
  Mux1/1 -> To Workspace1/1
  Product/1 -> Mux1/2  "Power"
  1 Ext on | -1 Ext off/1 -> Cylinder 1/5(Ext Control Input), Cylinder 2/5(Ext Control Input), Cylinder 3/5(Ext Control Input), Cylinder 4/5(Ext Control Input)
  1 Comp on | -1 Comp off/1 -> Cylinder 1/6(Comp Control Input), Cylinder 2/6(Comp Control Input), Cylinder 3/6(Comp Control Input), Cylinder 4/6(Comp Control Input)
  Sum2/1 -> PTO Force Scope1/1, Sum/1
  PS-Simulink Converter7/1 -> Mux/10  "Pressure Brine Exit"
  Discrete-Time Integrator/1 -> Accumulator Volume Scope/1
  PS-Simulink Converter/1 -> Discrete-Time Integrator/1
  PS-Simulink Converter9/1 -> Mux/9  "Brine Flow Rate"
  PS-Simulink Converter5/1 -> Mux/5  "Feed Pressure"
  Cylinder 1/1(PTO Force) -> Sum2/4
  PS-Simulink Converter8/1 -> Mux/8  "Permeate Mass Flow Rate"
  PS-Simulink Converter10/1 -> Mux/6  "Brine Mass Flow Rate"
  PS-Simulink Converter6/1 -> Mux/7  "Feed Mass Flow Rate"
  PS-Simulink Converter4/1 -> Mux/4  "Permeate Flow Rate"
  PS-Simulink Converter1/1 -> Mux/1  "P before RO after OSM"
  Constant1/1 -> Switch/3
  Mux/1 -> To Workspace/1
  Cylinder 2/1(PTO Force) -> Sum2/3
  Crank Radius (m)/1 -> Cylinder 1/1(Crank Radius), Cylinder 2/1(Crank Radius), Cylinder 3/1(Crank Radius), Cylinder 4/1(Crank Radius)
  PS-Simulink Converter2/1 -> Mux/2  "P drop RO"
  Ang Velocity signal/1 -> Discrete-Time Integrator - Angle Disp/1, Simulink-PS Converter/1
  Spool Radius (m)/1 -> Cylinder 1/2(Spool Radius), Cylinder 4/2(Spool Radius), Cylinder 3/2(Spool Radius), Cylinder 2/2(Spool Radius), Ang Velocity signal/2
  Discrete-Time Integrator - Angle Disp/1 -> Cylinder 4/3(Angle Displacement), Cylinder 3/3(Angle Displacement), Cylinder 2/3(Angle Displacement), Cylinder 1/3(Angle Displacement)
  Cylinder 4/1(PTO Force) -> Sum2/1
  Crank Initial Angle (rad) 3/1 -> Cylinder 3/4(Crank Init Angle)
  Crank Initial Angle (rad) 2/1 -> Cylinder 2/4(Crank Init Angle)
  Crank Initial Angle (rad) 1/1 -> Cylinder 1/4(Crank Init Angle)
  Cylinder 3/1(PTO Force) -> Sum2/2
  Switch/1 -> Ang Velocity signal/1
  Crank Initial Angle (rad) 4/1 -> Cylinder 4/4(Crank Init Angle)
  PS-Simulink Converter3/1 -> Mux/3  "Feed Flow Rate"
  connections:
  Hydraulic Reference/LConn1 -- 1000 psi Pressure Relief Valve/RConn1 -- Pressure Sensor RV/RConn1
  Water Quality Block/LConn4 -- RO Membrane/RConn4 -- PS-Simulink Converter4/LConn1
  Water Quality Block/LConn1 -- PS-Simulink Converter1/LConn1 -- RO Membrane/RConn1
  Cylinder 4/LConn1 -- Cylinder 3/LConn1 -- Cylinder 1/LConn1 -- Ideal Angular Velocity Source/LConn1 -- Cylinder 2/LConn1
  Water Quality Block/LConn3 -- PS-Simulink Converter3/LConn1 -- RO Membrane/RConn3
  Cylinder 1/LConn3 -- Cylinder 4/LConn3 -- Cylinder 3/LConn3 -- Cylinder 2/LConn3 -- Solver Configuration/RConn1 -- Ocean Intake (5m depth)/LConn1 -- Sea Water/RConn1
  Pressure Sensor RV/LConn1 -- 1000 psi Pressure Relief Valve/LConn1 -- RO Membrane/LConn1 -- Gas-Charged Accumulator/RConn1 -- Cylinder 1/LConn2 -- Cylinder 3/LConn2 -- Cylinder 4/LConn2 -- Cylinder 2/LConn2
  Water Quality Block/LConn2 -- PS-Simulink Converter2/LConn1 -- RO Membrane/RConn2
  PS-Simulink Converter10/LConn1 -- RO Membrane/RConn9
  PS-Simulink Converter8/LConn1 -- RO Membrane/RConn7
  PS-Simulink Converter7/LConn1 -- RO Membrane/RConn10
  RO Membrane/RConn5 -- PS-Simulink Converter5/LConn1
  Ideal Angular Velocity Source/RConn1 -- Simulink-PS Converter/RConn1
  PS-Simulink Converter9/LConn1 -- RO Membrane/RConn8
  PS-Simulink Converter6/LConn1 -- RO Membrane/RConn6
  Ideal Angular Velocity Source/RConn2 -- Mechanical Rotational Reference/LConn1
  " Flow Rate Accum Sensor"/RConn1 -- PS-Simulink Converter/LConn1

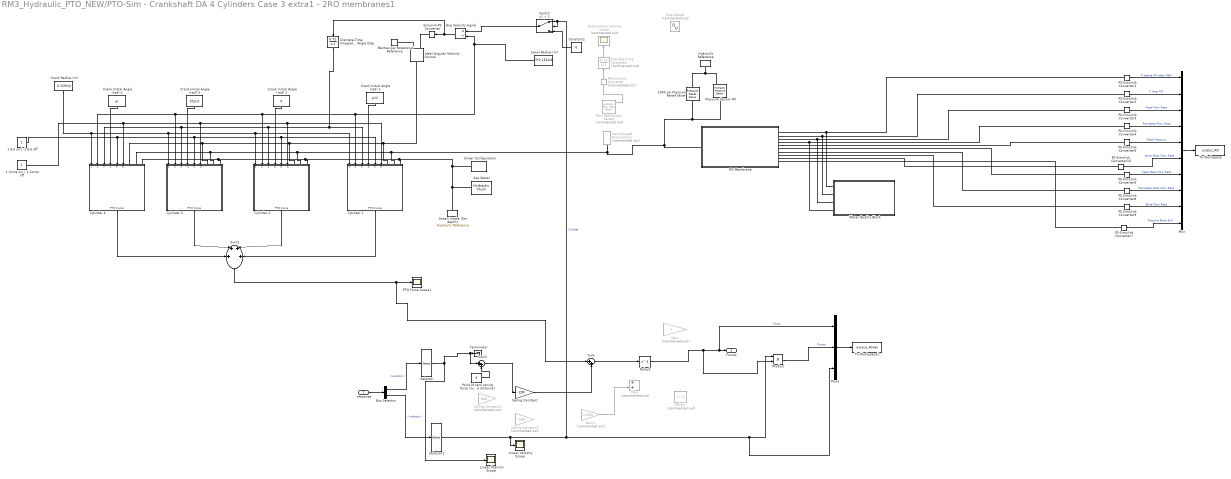
== system RM3_Hydraulic_PTO_NEW/PTO-Sim - Crankshaft DA 4 Cylinders Case 3 extra1 - 2RO membranes1 ==
  response : Inport
  " Flow Rate Accum Sensor" : fl_lib/Hydraulic/Hydraulic Sensors/Hydraulic Flow Rate Sensor  Commented=on
      settings: SourceProductName=Simscape
  1 Comp on | -1 Comp off : Constant
  1 Ext on | -1 Ext off : Constant
  1000 psi Pressure Relief Valve : sh_lib/Valves/Pressure Control Valves/Pressure Relief Valve  valve_area_spec=1  p_diff_TLU=[30.15e5 : 15e3 : 31.35e5] Pa  area_TLU=[1 : 1 : 9] .* 1e-5 m^2  area_max=pi*(0.75/2)^2 in^2  pres_set=1000 psi  reg_range=50 psi  C_d=0.7  A_leak=1e-12 m^2  lam_spec=1  B_lam=0.999  Re_cr=12  dynamic=0  tau=0.1 s  area_init=1e-12 m^2
      settings: SourceProductName=Simscape Fluids  SourceProductBaseCode=SH  InternalSimscapePortConfiguration="{\"Bottom\":[],\"Left\":[{\"id\":\"A\",\"label\":\"A\",\"type\":\"foundation.hydraulic.hydraulic\"}],\"Right\":[{\"id\":\"B\",\"label\":\"B\",\"type\":\"foundation.hydraulic.hydraulic\"}],\"Top\":[]}"
  Accumulator Volume Scope : Scope  Commented=on
  Ang Velocity signal : Product  Inputs=*/
  Bus Selector : BusSelector  OutputSignals=position,velocity
  Constant1 : Constant  Value=0
  Crank Initial Angle (rad) 1 : Constant  Value=pi/2
  Crank Initial Angle (rad) 2 : Constant  Value=0
  Crank Initial Angle (rad) 3 : Constant  Value=3*pi/2
  Crank Initial Angle (rad) 4 : Constant  Value=pi
  Crank Radius (m) : Constant  Value=0.1593/2
  Cylinder 1 : Subsystem
  Cylinder 2 : Subsystem
  Cylinder 3 : Subsystem
  Cylinder 4 : Subsystem
  Delay1 : Delay  Commented=on  DelayLength=1
  Delay2 : Delay  DelayLength=1
  Discrete-Time Integrator : DiscreteIntegrator  Commented=on  SampleTime=-1  ICPrevOutput=DiscIntNeverNeededParam  ICPrevScaledInput=DiscIntNeverNeededParam
  Discrete-Time Integrator - Angle Disp : DiscreteIntegrator  SampleTime=-1  ICPrevOutput=DiscIntNeverNeededParam  ICPrevScaledInput=DiscIntNeverNeededParam
  Gain : Gain  Commented=on
  Gain1 : Gain  Commented=on  Gain=-11000
  Gas-Charged Accumulator : sh_lib/Accumulators/Gas-Charged Accumulator  Commented=on  capacity=2.5 gal  dead_volume=4e-5 m^3  pr_preload=800 psi  k_sh=1.4  stiff_coeff=1e10 Pa/m^3  penetr_coeff=1e10 s*Pa/m^6  flow_rate_specify=off  flow_rate_priority=None  flow_rate=0.005 m^3/s  flow_rate_nominal_specify=off  flow_rate_nominal_unit=m^3/s  flow_rate_nominal_value=1  liquid_volume_specify=on  liquid_volume_priority=High  liquid_volume=0.005 m^3  liquid_volume_nominal_specify=off  liquid_volume_nominal_unit=m^3  liquid_volume_nominal_value=1  liquid_pressure_specify=off  liquid_pressure_priority=None  liquid_pressure=1.01325e+5 Pa  liquid_pressure_nominal_specify=off  liquid_pressure_nominal_unit=Pa  liquid_pressure_nominal_value=1
      settings: SourceProductName=Simscape Fluids  SourceProductBaseCode=SH  InternalSimscapePortConfiguration="{\"Bottom\":[],\"Left\":[],\"Right\":[{\"id\":\"A\",\"label\":\"A\",\"type\":\"foundation.hydraulic.hydraulic\"}],\"Top\":[]}"
  Hydraulic Reference : fl_lib/Hydraulic/Hydraulic Elements/Hydraulic Reference
      settings: SourceProductName=Simscape
  Ideal Angular Velocity Source : fl_lib/Mechanical/Mechanical Sources/Ideal Angular Velocity Source
  Linear Position Scope : Scope
  Linear Velocity Scope : Scope
  Mechanical Rotational Reference : fl_lib/Mechanical/Rotational Elements/Mechanical Rotational Reference
  Mux : Mux  Inputs=10
  Mux1 : Mux  Inputs=3
  Ocean Intake (5m depth) : fl_lib/Hydraulic/Hydraulic Elements/Hydraulic Reference
      settings: SourceProductName=Simscape
  PS-Simulink Converter : nesl_utility/PS-Simulink Converter  Commented=on  PhysicalDomain=network_engine_domain  SubClassName=ps_output  LeftPortType=input  RightPortType=output  PseudoPeriodic=off  Frequencies=[]  Unit=inherit  AffineConversion=off
  PS-Simulink Converter{1..10} (10 alike) : nesl_utility/PS-Simulink Converter  PhysicalDomain=network_engine_domain  SubClassName=ps_output  LeftPortType=input  RightPortType=output  PseudoPeriodic=off  Frequencies=[]  Unit=inherit  AffineConversion=off
  PTO Force Scope1 : Scope
  Plus : Sum  Commented=on
  "Point of zero spring force (submerged distance) " : Constant  Value=4
  Pressure Sensor RV : fl_lib/Hydraulic/Hydraulic Sensors/Hydraulic Pressure Sensor
      settings: SourceProductName=Simscape
  Product : Product
  RO Membrane : Subsystem
  Sea Water : sh_lib/Hydraulic Utilities/Hydraulic Fluid  DataSource=1  SelFluid=24  SysTemp=30  TrapAir=0.005  ViscDerFactor=1  range_error=2
      settings: SourceProductName=Simscape Fluids
  Selector : Selector  InputPortWidth=6  IndexOptions=Index vector (dialog)  Indices=3  OutputSizes=1
  Selector1 : Selector  InputPortWidth=6  IndexOptions=Index vector (dialog)  Indices=3  OutputSizes=1
  Simulink-PS Converter : nesl_utility/Simulink-PS Converter  PhysicalDomain=network_engine_domain  SubClassName=ps_input  LeftPortType=input  RightPortType=output  PseudoPeriodic=off  Frequencies=[]  NoiseDistribution=none  NoiseParameters=[]  Unit=rad/s  AffineConversion=off  FilteringAndDerivatives=filter  SimscapeFilterOrder=2  InputFilterTimeConstant=0.001  UdotUserProvided=0
  Sine Wave2 : Sin  Commented=on  Amplitude=0.45/4  Frequency=0.9  SampleTime=0.01
  Solver Configuration : nesl_utility/Solver Configuration  PhysicalDomain=network_engine_domain  SubClassName=solver  LeftPortType=input  RightPortType=generic  Tones=[]  Harmonics=[]  SimulateNoise=off  Profile=off  UseLocalSampling=off  EnableSwitchedLinearOptims=on  FrequencyDomain=off  UseCCode=off  RelTol=0.001  AbsTol=1e-06  MinStep=1e-09  ToWorkspace=off  RevertToSquareIcSolve=off  NumHomotopyIterations=100  PhasorMode=off  PhasorModeNumHarmonics=1  DoDC=off  ResidualTolerance=1e-09  UseLocalSolver=off  LocalSolverChoice=NE_BACKWARD_EULER_ADVANCER  LocalSolverSampleTime=0.001  DoFixedCost=off  MaxNonlinIter=3  MaxModeIter=2  LinearAlgebra=auto  EquationFormulation=NE_TIME_EF  DelaysMemoryBudget=1024  AutomaticFiltering=on  FilteringTimeConstant=0.01  PartitionStorageMethod=AS_NEEDED  PartitionMemoryBudget=1024  PartitionMethod=ROBUST
  Spool Radius (m) : Constant  Value=3*0.1520/4
  Spring Constant : Gain  Gain=-200
  Spring Constant1 : Gain  Commented=on  Gain=840
  Spring Constant2 : Gain  Commented=on  Gain=-400
  Sum : Sum  Inputs=|++
  Sum1 : Sum  Inputs=|++
  Sum2 : Sum  Inputs=4
  Switch : Switch  Criteria=u2 > Threshold
  Terminator : Terminator
  To Workspace : ToWorkspace  VariableName=output_RO  SaveFormat=Structure With Time  SampleTime=-1
  To Workspace1 : ToWorkspace  VariableName=output_Power  SaveFormat=Structure With Time  SampleTime=-1
  Water Quality Block : Subsystem
  Forces : Outport  VectorParamsAs1DForOutWhenUnconnected=off
  wires:
  Bus Selector/1 -> Selector/1  "<position>"
  Bus Selector/2 -> Selector1/1  "<velocity>"
  response/1 -> Bus Selector/1
  Selector/1 -> Linear Position Scope/1, Sum1/1, Terminator/1
  Spring Constant/1 -> Sum/2
  Gain1/1 -> Plus/2
  Sum/1 -> Delay2/1
  Selector1/1 -> Linear Velocity Scope/1, Mux1/3, Product/1, Switch/2, Switch/1  "V_linear"
  "Point of zero spring force (submerged distance) "/1 -> Sum1/2
  Sum1/1 -> Spring Constant/1
  Delay2/1 -> Product/2, Mux1/1, Forces/1  "Force"
  Mux1/1 -> To Workspace1/1
  Product/1 -> Mux1/2  "Power"
  1 Ext on | -1 Ext off/1 -> Cylinder 1/5(Ext Control Input), Cylinder 2/5(Ext Control Input), Cylinder 3/5(Ext Control Input), Cylinder 4/5(Ext Control Input)
  1 Comp on | -1 Comp off/1 -> Cylinder 1/6(Comp Control Input), Cylinder 2/6(Comp Control Input), Cylinder 3/6(Comp Control Input), Cylinder 4/6(Comp Control Input)
  Sum2/1 -> PTO Force Scope1/1, Sum/1
  PS-Simulink Converter7/1 -> Mux/10  "Pressure Brine Exit"
  Discrete-Time Integrator/1 -> Accumulator Volume Scope/1
  PS-Simulink Converter/1 -> Discrete-Time Integrator/1
  PS-Simulink Converter9/1 -> Mux/9  "Brine Flow Rate"
  PS-Simulink Converter5/1 -> Mux/5  "Feed Pressure"
  Cylinder 1/1(PTO Force) -> Sum2/4
  PS-Simulink Converter8/1 -> Mux/8  "Permeate Mass Flow Rate"
  PS-Simulink Converter10/1 -> Mux/6  "Brine Mass Flow Rate"
  PS-Simulink Converter6/1 -> Mux/7  "Feed Mass Flow Rate"
  PS-Simulink Converter4/1 -> Mux/4  "Permeate Flow Rate"
  PS-Simulink Converter1/1 -> Mux/1  "P before RO after OSM"
  Constant1/1 -> Switch/3
  Mux/1 -> To Workspace/1
  Cylinder 2/1(PTO Force) -> Sum2/3
  Crank Radius (m)/1 -> Cylinder 1/1(Crank Radius), Cylinder 2/1(Crank Radius), Cylinder 3/1(Crank Radius), Cylinder 4/1(Crank Radius)
  PS-Simulink Converter2/1 -> Mux/2  "P drop RO"
  Ang Velocity signal/1 -> Discrete-Time Integrator - Angle Disp/1, Simulink-PS Converter/1
  Spool Radius (m)/1 -> Cylinder 1/2(Spool Radius), Cylinder 4/2(Spool Radius), Cylinder 3/2(Spool Radius), Cylinder 2/2(Spool Radius), Ang Velocity signal/2
  Discrete-Time Integrator - Angle Disp/1 -> Cylinder 4/3(Angle Displacement), Cylinder 3/3(Angle Displacement), Cylinder 2/3(Angle Displacement), Cylinder 1/3(Angle Displacement)
  Cylinder 4/1(PTO Force) -> Sum2/1
  Crank Initial Angle (rad) 3/1 -> Cylinder 3/4(Crank Init Angle)
  Crank Initial Angle (rad) 2/1 -> Cylinder 2/4(Crank Init Angle)
  Crank Initial Angle (rad) 1/1 -> Cylinder 1/4(Crank Init Angle)
  Cylinder 3/1(PTO Force) -> Sum2/2
  Switch/1 -> Ang Velocity signal/1
  Crank Initial Angle (rad) 4/1 -> Cylinder 4/4(Crank Init Angle)
  PS-Simulink Converter3/1 -> Mux/3  "Feed Flow Rate"
  connections:
  Hydraulic Reference/LConn1 -- 1000 psi Pressure Relief Valve/RConn1 -- Pressure Sensor RV/RConn1
  Water Quality Block/LConn4 -- RO Membrane/RConn4 -- PS-Simulink Converter4/LConn1
  Water Quality Block/LConn1 -- PS-Simulink Converter1/LConn1 -- RO Membrane/RConn1
  Cylinder 4/LConn1 -- Cylinder 3/LConn1 -- Cylinder 1/LConn1 -- Ideal Angular Velocity Source/LConn1 -- Cylinder 2/LConn1
  Water Quality Block/LConn3 -- PS-Simulink Converter3/LConn1 -- RO Membrane/RConn3
  Cylinder 1/LConn3 -- Cylinder 4/LConn3 -- Cylinder 3/LConn3 -- Cylinder 2/LConn3 -- Solver Configuration/RConn1 -- Ocean Intake (5m depth)/LConn1 -- Sea Water/RConn1
  Pressure Sensor RV/LConn1 -- 1000 psi Pressure Relief Valve/LConn1 -- RO Membrane/LConn1 -- Gas-Charged Accumulator/RConn1 -- Cylinder 1/LConn2 -- Cylinder 3/LConn2 -- Cylinder 4/LConn2 -- Cylinder 2/LConn2
  Water Quality Block/LConn2 -- PS-Simulink Converter2/LConn1 -- RO Membrane/RConn2
  PS-Simulink Converter10/LConn1 -- RO Membrane/RConn9
  PS-Simulink Converter8/LConn1 -- RO Membrane/RConn7
  PS-Simulink Converter7/LConn1 -- RO Membrane/RConn10
  RO Membrane/RConn5 -- PS-Simulink Converter5/LConn1
  Ideal Angular Velocity Source/RConn1 -- Simulink-PS Converter/RConn1
  PS-Simulink Converter9/LConn1 -- RO Membrane/RConn8
  PS-Simulink Converter6/LConn1 -- RO Membrane/RConn6
  Ideal Angular Velocity Source/RConn2 -- Mechanical Rotational Reference/LConn1
  " Flow Rate Accum Sensor"/RConn1 -- PS-Simulink Converter/LConn1
